simulink subsystem "MPC4_nlpsol_ipopt"  (R2023b)
settings: Solver=VariableStepAuto  StartTime=0.0  StopTime=10.0  RelTol=1e-3
undefined symbols (not defined in the file): param_MPC4_ipopt_nlpsol, param_MPC4_ipopt_nlpsol_traj_data, param_weight_MPC4_ipopt_nlpsol
settings Model: Creator=emu  LastModifiedBy=emu

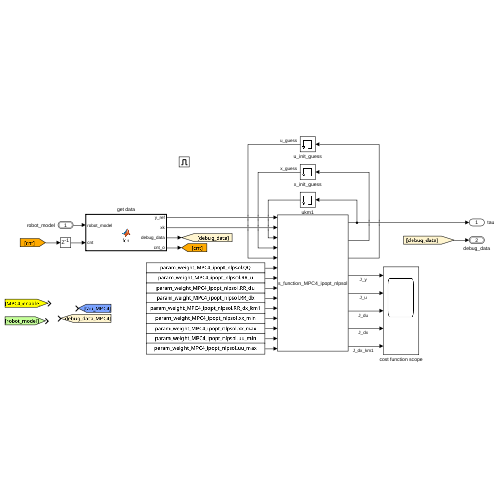
[thumbnail: Simulink's stored preview of the top-level diagram]
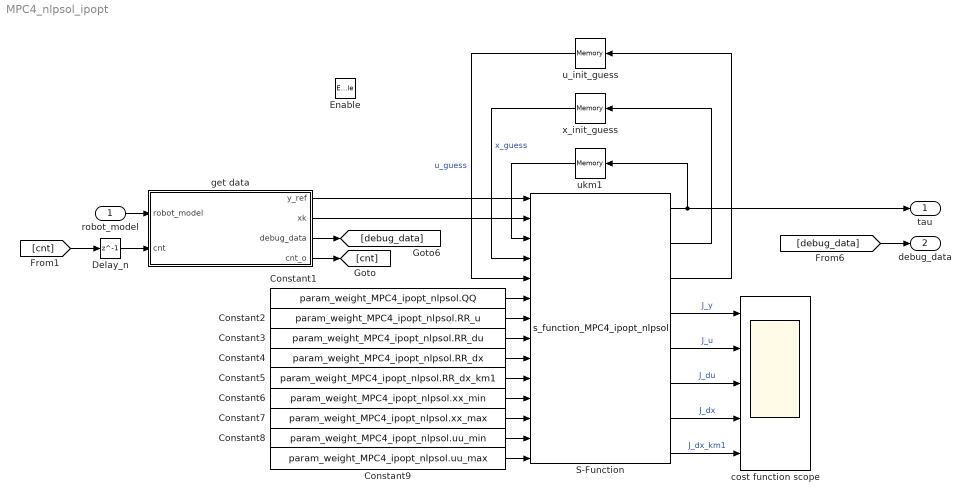
== system MPC4_nlpsol_ipopt ==
  robot_model : Inport  OutDataTypeStr=Bus: robot_model
  Enable : EnablePort
  Constant1 : Constant  Value=param_weight_MPC4_ipopt_nlpsol.QQ
  Constant2 : Constant  Value=param_weight_MPC4_ipopt_nlpsol.RR_u
  Constant3 : Constant  Value=param_weight_MPC4_ipopt_nlpsol.RR_du
  Constant4 : Constant  Value=param_weight_MPC4_ipopt_nlpsol.RR_dx
  Constant5 : Constant  Value=param_weight_MPC4_ipopt_nlpsol.RR_dx_km1
  Constant6 : Constant  Value=param_weight_MPC4_ipopt_nlpsol.xx_min
  Constant7 : Constant  Value=param_weight_MPC4_ipopt_nlpsol.xx_max
  Constant8 : Constant  Value=param_weight_MPC4_ipopt_nlpsol.uu_min
  Constant9 : Constant  Value=param_weight_MPC4_ipopt_nlpsol.uu_max
  Delay_n : Delay  DelayLength=1  InitialCondition=1
  S-Function : S-Function  FunctionName=s_function_MPC4_ipopt_nlpsol  Parameters='s_functions/MPC4_ipopt_nlpsol.casadi', 'MPC4_ipopt_nlpsol'  SFunctionDeploymentMode=off  EnableBusSupport=off
  cost function scope : Scope  NumInputPorts=5
  get data : MATLAB Function  TreatAsAtomicUnit=on
  u_init_guess : Memory  InitialCondition=param_MPC4_ipopt_nlpsol.u_init_guess
  ukm1 : Memory  InitialCondition=param_MPC4_ipopt_nlpsol.u_init_guess(:,1)
  x_init_guess : Memory  InitialCondition=param_MPC4_ipopt_nlpsol.x_init_guess
  tau : Outport
  debug_data : Outport  Port=2  OutDataTypeStr=Bus: debug_data_bus
  wires:
  Constant3/1 -> S-Function/8
  Delay_n/1 -> get data/2(cnt)
  Constant1/1 -> S-Function/6
  Constant8/1 -> S-Function/13
  S-Function/5 -> cost function scope/2  "J_u"
  Constant6/1 -> S-Function/11
  S-Function/3 -> u_init_guess/1
  get data/2(xk) -> S-Function/2
  [cnt] -> Delay_n/1
  get data/1(y_ref) -> S-Function/1
  Constant5/1 -> S-Function/10
  [debug_data] -> debug_data/1
  get data/3(debug_data) -> [debug_data]
  u_init_guess/1 -> S-Function/5  "u_guess"
  S-Function/7 -> cost function scope/4  "J_dx"
  S-Function/6 -> cost function scope/3  "J_du"
  S-Function/4 -> cost function scope/1  "J_y"
  S-Function/8 -> cost function scope/5  "J_dx_km1"
  Constant9/1 -> S-Function/14
  Constant2/1 -> S-Function/7
  x_init_guess/1 -> S-Function/4  "x_guess"
  Constant4/1 -> S-Function/9
  get data/4(cnt_o) -> [cnt]
  S-Function/1 -> ukm1/1, tau/1
  ukm1/1 -> S-Function/3
  S-Function/2 -> x_init_guess/1
  Constant7/1 -> S-Function/12
  robot_model/1 -> get data/1(robot_model)

== matlab function MPC4_nlpsol_ipopt/get data ==
  settings: updateMethod=DISCRETE  sampleTime=param_global.Ta
  data: y_ref output; robot_model input Bus: robot_model; cnt input; param_MPC4_ipopt_nlpsol parameter; xk output; debug_data output Bus: debug_data_bus; cnt_o output; param_MPC4_ipopt_nlpsol_traj_data parameter
function [y_ref, xk, debug_data, cnt_o] = fcn(robot_model, cnt, param_MPC4_ipopt_nlpsol, param_MPC4_ipopt_nlpsol_traj_data)

param_MPC = param_MPC4_ipopt_nlpsol;
N = param_MPC.N;
N_step = param_MPC.N_step;
param_trajectory = param_MPC4_ipopt_nlpsol_traj_data;

% Parameters
q = robot_model.q;      % generalized coordinates
q_p = robot_model.q_p;  % time derivative of generalized coordinates
H = robot_model.H;

% Current Pose of Endeffector
p = H(1:3,4);
R = H(1:3,1:3);

% desired Orientation as Rotationmatrix
q_e = rotation2quaternion(R);

% Error of Position (translation) and first time derivative
q_err = quat_mult(q_e, quat_inv(param_trajectory.q_d(:, cnt)));

xk = [q;q_p];

% Assemble vector of recieved output measurements
p_d_traj = param_trajectory.p_d(1:3, cnt: N_step : cnt + N*N_step);
y_ref = p_d_traj(1:2, 2:N+1);

cnt_o = cnt+1;

%% DEBUG
debug_data.x = p(1);
debug_data.x_d = p_d_traj(1,1);
debug_data.y =  p(2);
debug_data.y_d = p_d_traj(2,1);
debug_data.z =  p(3);
debug_data.z_d = p_d_traj(3,1);
debug_data.rot_x_err = q_err(2);
debug_data.rot_y_err = q_err(3);
debug_data.rot_z_err = q_err(4);
